simulink library "dcm"  (R2020b)
settings: Solver=VariableStepAuto  StartTime=0.0  StopTime=10.0  RelTol=1e-3
values from neighbouring files (symbols this model uses):
  A0 = eye(3)    [initial_conditions.m]
libraries: mat_3x3 x1
settings Model: Creator=whitehole  LastModifiedBy=whitehole

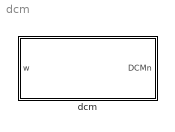
== system dcm ==
  dcm : Subsystem

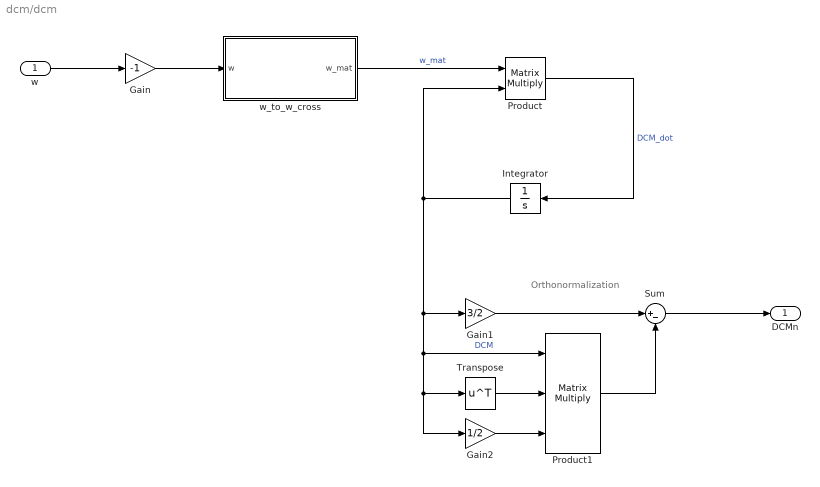
== system dcm/dcm ==
  note: Orthonormalization
  w : Inport
  Gain : Gain  Gain=-1
  Gain1 : Gain  Gain=3/2
  Gain2 : Gain  Gain=1/2
  Integrator : Integrator  InitialCondition=A0
  Product : Product  Multiplication=Matrix(*)
  Product1 : Product  Inputs=3  Multiplication=Matrix(*)
  Sum : Sum  Inputs=|+-
  Transpose : Math  Operator=transpose  SaturateOnIntegerOverflow=on
  w_to_w_cross : Subsystem
  DCMn : Outport
  wires:
  w/1 -> Gain/1
  Gain/1 -> w_to_w_cross/1(w)
  Product/1 -> Integrator/1  "DCM_dot"
  w_to_w_cross/1(w_mat) -> Product/1  "w_mat"
  Integrator/1 -> Product/2, Gain2/1, Transpose/1, Product1/1, Gain1/1  "DCM"
  Gain1/1 -> Sum/1
  Product1/1 -> Sum/2
  Gain2/1 -> Product1/3
  Transpose/1 -> Product1/2
  Sum/1 -> DCMn/1

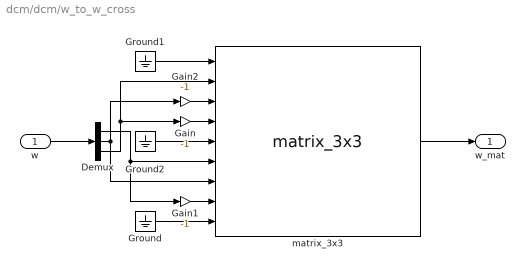
== system dcm/dcm/w_to_w_cross ==
  w : Inport
  Demux : Demux  Outputs=3
  Gain : Gain  Gain=-1
  Gain1 : Gain  Gain=-1
  Gain2 : Gain  Gain=-1
  Ground : Ground
  Ground1 : Ground
  Ground2 : Ground
  matrix_3x3 : mat_3x3/matrix_3x3  SystemSampleTime=-1  VariantActivationTime=update diagram  Latency=0  AutoFrameSizeCalculation=off
  w_mat : Outport
  wires:
  w/1 -> Demux/1
  matrix_3x3/1 -> w_mat/1
  Gain/1 -> matrix_3x3/4
  Gain1/1 -> matrix_3x3/8
  Gain2/1 -> matrix_3x3/3
  Demux/3 -> Gain/1, matrix_3x3/2
  Demux/2 -> matrix_3x3/7, Gain2/1
  Demux/1 -> matrix_3x3/6, Gain1/1
  Ground/1 -> matrix_3x3/9
  Ground1/1 -> matrix_3x3/1
  Ground2/1 -> matrix_3x3/5
